simulink model "simulation_Hippocampus_compare_paper"  (R2023a)
settings: Solver=ode3  StartTime=0  StopTime=120  FixedStep=0.001  MaxStep=0.001  MinStep=0.00001  RelTol=1e-5  AbsTol=1e-5  EnableMultiTasking=on
values from neighbouring files (symbols this model uses):
  k_pos_ndi = 8    [parameters.m]
  k_vel_ndi = 8    [parameters.m]
  Kf = 6    [parameters.m]
  Kp = 0.01    [parameters.m]
  Kp_p = 30    [parameters.m]
  Kp_pitch = 8    [parameters.m]
  Kp_q = 10    [parameters.m]
  Kp_r = 10    [parameters.m]
  Kp_roll = 10    [parameters.m]
  Kp_u = 8    [parameters.m]
  Kp_yaw = 8    [parameters.m]
  Kq = 5    [parameters.m]
  Kr = 8    [parameters.m]
  Ktau1 = 0.1    [parameters.m]
  Ktau2 = 5    [parameters.m]
  Ktau3 = 5    [parameters.m]
  Ku = 8    [parameters.m]
  p11 = 0.4    [parameters.m]
  p12 = 0.2    [parameters.m]
  p21 = 0.2    [parameters.m]
  p22 = 0.05    [parameters.m]
  p31 = 0.3    [parameters.m]
  p32 = 0.05    [parameters.m]
  p41 = 0.5    [parameters.m]
  p42 = 0.1    [parameters.m]
  p51 = 0.5    [parameters.m]
  p52 = 0.1    [parameters.m]
  p61 = 0.5    [parameters.m]
  p62 = 0.1    [parameters.m]
  Q1 = -8    [simulation_para.m]
  Q2 = -10    [simulation_para.m]
  Q3 = -[0.01,5,8]    [simulation_para.m]
  Q4 = -[0.001,0.1,0.1]    [simulation_para.m]
  r1 = 4    [parameters.m]
  r2 = 6    [parameters.m]
libraries: simulink x8
(part 4 of 7)

== system simulation_Hippocampus_compare_paper/NDI4/Disturbance: All derivatives2/disturbance3/Subsystem1/wave frenquency ==
  Constant2 : Constant
  Constant3 : Constant  Value=1.1
  Constant4 : Constant  Value=1.2
  Constant5 : Constant  Value=0.5
  Constant6 : Constant  Value=0.6
  Constant7 : Constant  Value=0.7
  Mux : Mux  Inputs=6
  Out1 : Outport
  wires:
  Constant3/1 -> Mux/2
  Constant2/1 -> Mux/1
  Constant4/1 -> Mux/3
  Constant7/1 -> Mux/6
  Mux/1 -> Out1/1
  Constant5/1 -> Mux/4
  Constant6/1 -> Mux/5

== system simulation_Hippocampus_compare_paper/NDI4/Disturbance: All derivatives2/disturbance3/Subsystem1/wave percentage ==
  Constant{2..7} (6 alike) : Constant  Value=0
  Mux : Mux  Inputs=6
  Out1 : Outport
  wires:
  Constant3/1 -> Mux/2
  Constant2/1 -> Mux/1
  Constant4/1 -> Mux/3
  Constant7/1 -> Mux/6
  Mux/1 -> Out1/1
  Constant5/1 -> Mux/4
  Constant6/1 -> Mux/5

== system simulation_Hippocampus_compare_paper/PDPD/Disturbance: All derivatives1/disturbance3/Subsystem1/wave frenquency ==
  Constant2 : Constant
  Constant3 : Constant  Value=1.1
  Constant4 : Constant  Value=1.2
  Constant5 : Constant  Value=0.5
  Constant6 : Constant  Value=0.6
  Constant7 : Constant  Value=0.7
  Mux : Mux  Inputs=6
  Out1 : Outport
  wires:
  Constant3/1 -> Mux/2
  Constant2/1 -> Mux/1
  Constant4/1 -> Mux/3
  Constant7/1 -> Mux/6
  Mux/1 -> Out1/1
  Constant5/1 -> Mux/4
  Constant6/1 -> Mux/5

== system simulation_Hippocampus_compare_paper/PDPD/Disturbance: All derivatives1/disturbance3/Subsystem1/wave percentage ==
  Constant{2..7} (6 alike) : Constant  Value=0
  Mux : Mux  Inputs=6
  Out1 : Outport
  wires:
  Constant3/1 -> Mux/2
  Constant2/1 -> Mux/1
  Constant4/1 -> Mux/3
  Constant7/1 -> Mux/6
  Mux/1 -> Out1/1
  Constant5/1 -> Mux/4
  Constant6/1 -> Mux/5

== system simulation_Hippocampus_compare_paper/PDPD1/Disturbance: All derivatives1/disturbance3/Subsystem1/wave frenquency ==
  Constant2 : Constant
  Constant3 : Constant  Value=1.1
  Constant4 : Constant  Value=1.2
  Constant5 : Constant  Value=0.5
  Constant6 : Constant  Value=0.6
  Constant7 : Constant  Value=0.7
  Mux : Mux  Inputs=6
  Out1 : Outport
  wires:
  Constant3/1 -> Mux/2
  Constant2/1 -> Mux/1
  Constant4/1 -> Mux/3
  Constant7/1 -> Mux/6
  Mux/1 -> Out1/1
  Constant5/1 -> Mux/4
  Constant6/1 -> Mux/5

== system simulation_Hippocampus_compare_paper/PDPD1/Disturbance: All derivatives1/disturbance3/Subsystem1/wave percentage ==
  Constant{2..7} (6 alike) : Constant  Value=0
  Mux : Mux  Inputs=6
  Out1 : Outport
  wires:
  Constant3/1 -> Mux/2
  Constant2/1 -> Mux/1
  Constant4/1 -> Mux/3
  Constant7/1 -> Mux/6
  Mux/1 -> Out1/1
  Constant5/1 -> Mux/4
  Constant6/1 -> Mux/5

== system simulation_Hippocampus_compare_paper/Proposed Linear gain/Disturbance: All derivatives1/disturbance3/Subsystem1/wave frenquency ==
  Constant2 : Constant
  Constant3 : Constant  Value=1.1
  Constant4 : Constant  Value=1.2
  Constant5 : Constant  Value=0.5
  Constant6 : Constant  Value=0.6
  Constant7 : Constant  Value=0.7
  Mux : Mux  Inputs=6
  Out1 : Outport
  wires:
  Constant3/1 -> Mux/2
  Constant2/1 -> Mux/1
  Constant4/1 -> Mux/3
  Constant7/1 -> Mux/6
  Mux/1 -> Out1/1
  Constant5/1 -> Mux/4
  Constant6/1 -> Mux/5

== system simulation_Hippocampus_compare_paper/Proposed Linear gain/Disturbance: All derivatives1/disturbance3/Subsystem1/wave percentage ==
  Constant{2..7} (6 alike) : Constant  Value=0
  Mux : Mux  Inputs=6
  Out1 : Outport
  wires:
  Constant3/1 -> Mux/2
  Constant2/1 -> Mux/1
  Constant4/1 -> Mux/3
  Constant7/1 -> Mux/6
  Mux/1 -> Out1/1
  Constant5/1 -> Mux/4
  Constant6/1 -> Mux/5

== system simulation_Hippocampus_compare_paper/Proposed Linear gain/Disturbance: All derivatives2/disturbance3/Subsystem1/wave frenquency ==
  Constant2 : Constant
  Constant3 : Constant  Value=1.1
  Constant4 : Constant  Value=1.2
  Constant5 : Constant  Value=0.5
  Constant6 : Constant  Value=0.6
  Constant7 : Constant  Value=0.7
  Mux : Mux  Inputs=6
  Out1 : Outport
  wires:
  Constant3/1 -> Mux/2
  Constant2/1 -> Mux/1
  Constant4/1 -> Mux/3
  Constant7/1 -> Mux/6
  Mux/1 -> Out1/1
  Constant5/1 -> Mux/4
  Constant6/1 -> Mux/5

== system simulation_Hippocampus_compare_paper/Proposed Linear gain/Disturbance: All derivatives2/disturbance3/Subsystem1/wave percentage ==
  Constant{2..7} (6 alike) : Constant  Value=0
  Mux : Mux  Inputs=6
  Out1 : Outport
  wires:
  Constant3/1 -> Mux/2
  Constant2/1 -> Mux/1
  Constant4/1 -> Mux/3
  Constant7/1 -> Mux/6
  Mux/1 -> Out1/1
  Constant5/1 -> Mux/4
  Constant6/1 -> Mux/5

== system simulation_Hippocampus_compare_paper/Proposed Linear gain1/Disturbance: All derivatives1/disturbance3/Subsystem1/wave frenquency ==
  Constant2 : Constant
  Constant3 : Constant  Value=1.1
  Constant4 : Constant  Value=1.2
  Constant5 : Constant  Value=0.5
  Constant6 : Constant  Value=0.6
  Constant7 : Constant  Value=0.7
  Mux : Mux  Inputs=6
  Out1 : Outport
  wires:
  Constant3/1 -> Mux/2
  Constant2/1 -> Mux/1
  Constant4/1 -> Mux/3
  Constant7/1 -> Mux/6
  Mux/1 -> Out1/1
  Constant5/1 -> Mux/4
  Constant6/1 -> Mux/5

== system simulation_Hippocampus_compare_paper/Proposed Linear gain1/Disturbance: All derivatives1/disturbance3/Subsystem1/wave percentage ==
  Constant{2..7} (6 alike) : Constant  Value=0
  Mux : Mux  Inputs=6
  Out1 : Outport
  wires:
  Constant3/1 -> Mux/2
  Constant2/1 -> Mux/1
  Constant4/1 -> Mux/3
  Constant7/1 -> Mux/6
  Mux/1 -> Out1/1
  Constant5/1 -> Mux/4
  Constant6/1 -> Mux/5

== system simulation_Hippocampus_compare_paper/Proposed nonlinear gain/Disturbance: All derivatives1/disturbance3/Subsystem1/wave frenquency ==
  Constant2 : Constant
  Constant3 : Constant  Value=1.1
  Constant4 : Constant  Value=1.2
  Constant5 : Constant  Value=0.5
  Constant6 : Constant  Value=0.6
  Constant7 : Constant  Value=0.7
  Mux : Mux  Inputs=6
  Out1 : Outport
  wires:
  Constant3/1 -> Mux/2
  Constant2/1 -> Mux/1
  Constant4/1 -> Mux/3
  Constant7/1 -> Mux/6
  Mux/1 -> Out1/1
  Constant5/1 -> Mux/4
  Constant6/1 -> Mux/5

== system simulation_Hippocampus_compare_paper/Proposed nonlinear gain/Disturbance: All derivatives1/disturbance3/Subsystem1/wave percentage ==
  Constant{2..7} (6 alike) : Constant  Value=0
  Mux : Mux  Inputs=6
  Out1 : Outport
  wires:
  Constant3/1 -> Mux/2
  Constant2/1 -> Mux/1
  Constant4/1 -> Mux/3
  Constant7/1 -> Mux/6
  Mux/1 -> Out1/1
  Constant5/1 -> Mux/4
  Constant6/1 -> Mux/5

== system simulation_Hippocampus_compare_paper/Proposed nonlinear gain1/Disturbance: All derivatives1/disturbance3/Subsystem1/wave frenquency ==
  Constant2 : Constant
  Constant3 : Constant  Value=1.1
  Constant4 : Constant  Value=1.2
  Constant5 : Constant  Value=0.5
  Constant6 : Constant  Value=0.6
  Constant7 : Constant  Value=0.7
  Mux : Mux  Inputs=6
  Out1 : Outport
  wires:
  Constant3/1 -> Mux/2
  Constant2/1 -> Mux/1
  Constant4/1 -> Mux/3
  Constant7/1 -> Mux/6
  Mux/1 -> Out1/1
  Constant5/1 -> Mux/4
  Constant6/1 -> Mux/5

== system simulation_Hippocampus_compare_paper/Proposed nonlinear gain1/Disturbance: All derivatives1/disturbance3/Subsystem1/wave percentage ==
  Constant{2..7} (6 alike) : Constant  Value=0
  Mux : Mux  Inputs=6
  Out1 : Outport
  wires:
  Constant3/1 -> Mux/2
  Constant2/1 -> Mux/1
  Constant4/1 -> Mux/3
  Constant7/1 -> Mux/6
  Mux/1 -> Out1/1
  Constant5/1 -> Mux/4
  Constant6/1 -> Mux/5

== matlab function simulation_Hippocampus_compare_paper/Proposed Linear gain1/HippCampus/Subsystem1/norm1 ==
  data: u input; y output
function y  = fcn(u)
y=norm(u)^2;
end

== matlab function simulation_Hippocampus_compare_paper/Proposed Linear gain1/HippCampus/Subsystem4/Subsystem/norm1 ==
  data: u input; y output
function y  = fcn(u)
y=norm(u)^2;
end

== matlab function simulation_Hippocampus_compare_paper/Proposed Linear gain1/HippCampus/Subsystem4/Subsystem1/norm1 ==
  data: u input; y output
function y  = fcn(u)
y=norm(u)^2;
end

== matlab function simulation_Hippocampus_compare_paper/Proposed Linear gain1/HippCampus/Subsystem4/Subsystem2/norm1 ==
  data: u input; y output
function y  = fcn(u)
y=norm(u)^2;
end

== matlab function simulation_Hippocampus_compare_paper/Proposed Linear gain1/HippCampus/Subsystem4/Subsystem3/norm1 ==
  data: u input; y output
function y  = fcn(u)
y=norm(u)^2;
end

== matlab function simulation_Hippocampus_compare_paper/Proposed nonlinear gain1/Controller/MATLAB Function1 ==
  data: ref input; K output; s input; k input; parameter input
%---------------------------------------------------------------------------------------------
% For Paper, 
% "Three-Dimensional Simultaneous Stabilization and Tracking Control of Nonholonomic Autonomous Underwater Vehicles"
% by Shuyuan Fan and Herbert Werner
% Copyright (c) Institute of Control Systems, Hamburg University of Technology. All rights reserved.
% Licensed under the GPLv3. See LICENSE in the project root for license information.
% Uses an own implementation of the work of 
% IEEE Conference on Decision and Control and L-CSS, 2022."
% Author(s): Shuyuan Fan
%--------------------------------------------------------------------------------------------
function K= fcn(ref,s,k,parameter)


%% reference
x_ref = ref(1);y_ref = ref(2);z_ref = ref(3);

%% states
x = s(1);y = s(2);z = s(3);
phi = s(4); phi =min(max(phi,-0.5),0.5);
theta = s(5); 
theta = min(max(theta,-1.5),1.5);
psi = s(6); psi =  wrapToPi(psi);
u=s(7);v=s(8);w=s(9); p =s(10);
q=s(11);r=s(12);

%% error
e_x = x_ref-x;
e_y = y_ref - y;
e_z = z_ref - z;

%% design attitude trajectory
psi_des = atan2(e_y, e_x);
e_psi = psi_des -psi;
e_psi = atan2(sin(e_psi), cos(e_psi));

theta_des = -atan2(e_z,(e_x^2+e_y^2)^0.5);
theta_des = min(max(theta_des,-1.5),1.5);
e_theta = theta_des - theta;

e_phi=0-phi;

%% gain
K0 =k(1);
K1 =k(2);
K2 =k(3);
K3 =k(4);

%% nonlinear gain
a1 = e_x^2 + e_y^2 + e_z^2;
a2=(e_x^2+e_y^2)^0.5;
p11 = parameter(1);
p12 = parameter(2);
p21 = parameter(3);
p22 = parameter(4);
p31 = parameter(5);
p32 = parameter(6);
e1 = e_x*cos(theta)*cos(psi)+e_y*cos(theta)*sin(psi)-e_z * sin(theta);
K0 = K0*(sqrt(a1)+p11)/(sqrt(a1)+p12);
K2 = K2*(abs(e_theta)+p21)/(abs(e_theta)+p22);
K3 = K3*(1*abs(e_psi)+p31)/(abs(e_psi)+p32);

% K0 = K0*(sqrt(a1)+0.4)/(sqrt(a1)+0.1);
% K2 = K2*(abs(e_theta)+0.2)/(abs(e_theta)+0.1);
% K3 = K3*(1*abs(e_psi)+0.5)/(abs(e_psi)+0.2);

%% design u

ud = K0*e1;

%% calculate exdot,eydot,ezdot

R =- [  cos(psi)*cos(theta)  cos(psi)*sin(theta)*sin(phi)-sin(psi)*cos(phi)  cos(psi)*cos(phi)*sin(theta)+sin(psi)*sin(phi) ;
           sin(psi)*cos(theta)  sin(psi)*sin(theta)*sin(phi)+cos(psi)*cos(phi)  sin(psi)*cos(phi)*sin(theta)-cos(psi)*sin(phi) ;
          -sin(theta)           cos(theta)*sin(phi)                             cos(theta)*cos(phi)                            ];

ee=R*[u;v;w];
exdot=ee(1);
eydot=ee(2);
ezdot=ee(3);


%% calculate theta_d_dot psi_d_dot
% % because atan2 is not continued and its derivative is not existing 
if abs(e_x)+abs(e_y)==0
%if  norm(e_x)+ norm(e_y) + norm(e_z) ==0 || norm(e_x)+ norm(e_y)==0
  theta_des_dot =0;
else
    theta_des_dot= -(ezdot*a2^2-2*e_z*(e_x*exdot+e_y*eydot))/(a1*a2+eps);
end

if abs(e_x)+abs(e_y)==0
    psi_des_dot = 0;
else
   psi_des_dot = (eydot*(e_x)-exdot*e_y)/((e_x)^2+e_y^2+eps);
end

 theta_des_dot = min(max(theta_des_dot,-3),3);
 psi_des_dot = min(max(psi_des_dot,-3),3);


%% design pd qd rd

pd = K1*e_phi-sin(phi)*tan(theta)*q-cos(phi)*tan(theta)*r;
qd = (K2*e_theta +r*sin(phi)+theta_des_dot)/(cos(phi)+eps);
rd = cos(theta)/(cos(phi)+eps)*(K3*e_psi+1*psi_des_dot-q*sin(phi)/(cos(theta)+eps));


%% saturation 
% ud=min(max(ud,-10),10);
% pd=min(max(pd,-6),6);
% qd=min(max(qd,-6),6);
% rd=min(max(rd,-10),10);

K = [ud;pd;qd;rd;e1;e_phi;e_theta;e_psi;theta_des_dot;psi_des_dot];
end

== matlab function simulation_Hippocampus_compare_paper/Stabilizing without v w /Controller/Kinematic1 ==
  data: sd input; s input; output output; sd_dot input; error1 input; k2 input
%---------------------------------------------------------------------------------------------
% For Paper, 
% "Three-Dimensional Simultaneous Stabilization and Tracking Control of Nonholonomic Autonomous Underwater Vehicles"
% by Shuyuan Fan and Herbert Werner
% Copyright (c) Institute of Control Systems, Hamburg University of Technology. All rights reserved.
% Licensed under the GPLv3. See LICENSE in the project root for license information.
% Uses an own implementation of the work of 
% IEEE Conference on Decision and Control and L-CSS, 2022."
% Author(s): Shuyuan Fan
%--------------------------------------------------------------------------------------------
function output = fcn(sd,s,sd_dot,error1,k2)  
    zg    =  0.05;    % [m]
    g     =  9.81;    % [m/s^2]

    m     =  1.43;    % [kg]
    Ix    = 0.00241; % [kgm^2]
    Iy    = 0.01072; % [kgm^2]
    Iz    = 0.01072; % [kgm^2]
    Xudot = -1.11;    % [kg]
    Yvdot = -2.80;    % [kg]
    Zwdot = -2.80;    % [kg]
    Kpdot = -0.0018;  % [kgm^2]
    Mqdot = -0.0095;  % [kgm^2]
    Nrdot = -0.0095;  % [kgm^2]
    Xu    = -4.56;    % [kg/m]
    Yv    = -17.36;   % [kg/m]
    Zw    = -17.36;   % [kg/m]
    Kp    = -0.0028;  % [kgm^2]
    Mq    = -0.0476;  % [kgm^2]
    Nr    = -0.0476;  % [kgm^2]

    udes = sd(1); pdes = sd(2);qdes=sd(3);rdes=sd(4);
    x=s;
    
    udes_dot=sd_dot(1);pd_dot =sd_dot(2);qd_dot = sd_dot(3);
    rd_dot = sd_dot(4); 
    
    e1 = error1(1);e_phi = error1(2);e_theta= error1(3);
    e_psi = error1(4);

    % Extract states into more readable form
    phi = x( 4); theta = x(5); psi = x( 6);
    u   = x( 7); v     = x( 8); w   = x( 9);
    p   = x(10); q     = x(11); r   = x(12);
    nu  = x(7:12);
    theta = min(max(theta,-1.5),1.5);
    % Construct rotational tensor
  R = [  cos(psi)*cos(theta)  cos(psi)*sin(theta)*sin(phi)-sin(psi)*cos(phi)  cos(psi)*cos(phi)*sin(theta)+sin(psi)*sin(phi) ;
   sin(psi)*cos(theta)  sin(psi)*sin(theta)*sin(phi)+cos(psi)*cos(phi)  sin(psi)*cos(phi)*sin(theta)-cos(psi)*sin(phi) ;
  -sin(theta)           cos(theta)*sin(phi)                            cos(theta)*cos(phi)                            ];


    % Construct velocity transformation tensor
    T = [ 1  sin(phi)*tan(theta)   cos(phi)*tan(theta) ;
          0  cos(phi)             -sin(phi)            ;
          0  sin(phi)/cos(theta)   cos(phi)/cos(theta) ];
    J = blkdiag(R, T);

    % Calculate mass matrix
    Ma  = -blkdiag(Xudot, Yvdot, Zwdot, Kpdot, Mqdot, Nrdot);
    Mrb =  blkdiag(eye(3) * m, Ix, Iy, Iz);
    M = Ma + Mrb;

    % Compute hydrostatic load
    gravity = zg * g * m;
    G = blkdiag(0,0,0, gravity * cos(theta) * (sin(phi)/(phi+eps)), gravity * (sin(theta)/(theta+eps)), 0);

    % Construct coriolis matrix, see Fossen 2011, Theorem 3.2
    C = [  zeros(3)                    -skew(M(1:3,1:3) * nu(1:3)) ;
          -skew(M(1:3,1:3) * nu(1:3))  -skew(M(4:6,4:6) * nu(4:6)) ];

    % Construct damping matrix
    D = -blkdiag(Xu * abs(u), Yv * abs(v),...
                 Zw * abs(w), Kp * abs(p),...
                 Mq * abs(q), Nr * abs(r));

    % Build state space equations
    
    Mi  = inv(M);
    A   = [ zeros(6), J; -Mi*G, -Mi*(C+D) ];
     
    dx  = A * x ;
    udot = dx(7);
    pdot = dx(10);
    qdot = dx(11);
    rdot = dx(12);
    
%%gain   

Kf =k2(1);
K_t1 =k2(2);
K_t2 =k2(3);
K_t3 =k2(4);


%% error2
eu = udes-u;
ep =pdes-p;
eq = qdes-q;
er = rdes-r;


%% nonlinear gain
% Kf=(1*abs(eu)+0.4)/(1*abs(eu)+0.11)*Kf;
% %K_t1 = (1*abs(ep)+0.15)/(1*abs(ep)+0.1)*K_t1;
% K_t2 = (1*abs(eq)+0.5)/(1*abs(eq)+0.1)*K_t2;
% K_t3 = (1*abs(er)+0.5)/(1*abs(er)+0.1)*K_t3;



%% controller
f=Kf*eu-udot*(m-Xudot)+udes_dot*(m-Xudot)+(m-Xudot)*e1;
tau1 = K_t1 * ep+0*(Ix-Kpdot)*(e_phi+pd_dot-pdot);
tau2 = K_t2 * eq  +(qd_dot+cos(phi)*e_theta-qdot)*(Iy-Mqdot);
tau3 = K_t3* er +(rd_dot+cos(phi)/(cos(theta)+eps)*e_psi-rdot)*(Iz-Nrdot);

controller =  [f;tau1;tau2;tau3];
error2 =[eu;ep;eq;er];

output = [controller;error2];



   

end
function S = skew(lambda)
    S = [  0          -lambda(3)   lambda(2) ;
           lambda(3)   0          -lambda(1) ;
          -lambda(2)   lambda(1)   0         ]; 
end

== matlab function simulation_Hippocampus_compare_paper/Proposed Linear gain1/norm ==
  data: u input; y output
function y  = fcn(u)
y=norm(u)^2;
end

== matlab function simulation_Hippocampus_compare_paper/Proposed Linear gain1/norm1 ==
  data: u input; y output
function y  = fcn(u)
y=norm(u);
end

== matlab function simulation_Hippocampus_compare_paper/Proposed nonlinear gain1/Controller/calculate derivative 1/MATLAB Function ==
  data: u input; y output; t input
function y = fcn(u,t)
if t>0.1
    y=u;
else
    y=[0;0;0;0];
end

== matlab function simulation_Hippocampus_compare_paper/Proposed nonlinear gain1/Disturbance: All derivatives1/MATLAB Function ==
  data: u input; y output; d input
function y = fcn(u,d)

y = u*d;

== matlab function simulation_Hippocampus_compare_paper/Proposed nonlinear gain1/Disturbance: All derivatives1/disturbance3/MATLAB Function ==
  data: p input; a input; d output; u_wave input; u_c input; u_un input
%% wind disturbance, wave disturbance, ocean currents and modeling uncertainties(Fossen 2011)
%for AUV, we can neglect the wind disturbance
%wave disturbance is in R^6
%Ocean Currents are related to the hydrodynamic terms. Here we consider
%them as the friction forces 
%modeling uncertainties can be assumed as constant terms
%assume all disturbances are constant
function d = fcn(p,a,u_wave, u_c,u_un)
%a: attitude states
%u_wave: parameters of u_wave
%u_c ocean currents percentage
%u_un uncertainty percentage
%ocean currents
phi=a(1);
theta=a(2);
psi = a(3);
V = u_c(1)/100*4.724; % 0<V<4.724
theta_c=u_c(2);
psi_c = u_c(3);
 R = [  cos(psi)*cos(theta)  cos(psi)*sin(theta)*sin(phi)-sin(psi)*cos(phi)  cos(psi)*cos(phi)*sin(theta)+sin(psi)*sin(phi) ;
           sin(psi)*cos(theta)  sin(psi)*sin(theta)*sin(phi)+cos(psi)*cos(phi)  sin(psi)*cos(phi)*sin(theta)-cos(psi)*sin(phi) ;
          -sin(theta)           cos(theta)*sin(phi)                             cos(theta)*cos(phi)                            ];
uc=[V*cos(theta_c)*cos(psi_c);V*sin(psi_c);V*sin(theta_c)*cos(psi_c)];
f_c=R*uc;
d_c=[f_c;zeros(3,1)];

%wave disturbance
k1=u_wave(1:6); %amplitude 
k2 = u_wave(7:12); %frequency 
time=u_wave(13);
d_w = [k1(1)/100*4.724*sin(k2(1)*time);k1(2)/100*4.724*sin(k2(2)*time);k1(3)/100*4.724*sin(k2(3)*time);
    k1(4)/100*6.841*sin(k2(4)*time);k1(5)/100*28.55*sin(k2(5)*time);k1(6)/100*28.55*sin(k2(6)*time)];
%model uncertainties
%u_un uncertainty percentage
d_u=u_un/100*[4.724;0;0;6.841;28.55;28.55];

x=p(1);
y=p(2);
z=p(3);
if y>2 && y<2.5 || y<-2 && y>-2.5
    tau_d=d_c+d_w+d_u;
else
    tau_d=zeros(6,1);
end
    
d=[zeros(6,1);tau_d];

== matlab function simulation_Hippocampus_compare_paper/Proposed nonlinear gain1/HippCampus/HippoCampus ==
  data: x input; dx output; in input
function dx = fcn(x, in)
zg    =  0.05;    % [m]
g     =  9.81;    % [m/s^2]

m     =  1.43;    % [kg]
Ix    = 0.00241; % [kgm^2]
Iy    = 0.01072; % [kgm^2]
Iz    = 0.01072; % [kgm^2]
Xudot = -1.11;    % [kg]
Yvdot = -2.80;    % [kg]
Zwdot = -2.80;    % [kg]
Kpdot = -0.0018;  % [kgm^2]
Mqdot = -0.0095;  % [kgm^2]
Nrdot = -0.0095;  % [kgm^2]
Xu    = -4.56;    % [kg/m]
Yv    = -17.36;   % [kg/m]
Zw    = -17.36;   % [kg/m]
Kp    = -0.0028;  % [kgm^2]
Mq    = -0.0476;  % [kgm^2]
Nr    = -0.0476;  % [kgm^2]
% Extract states into more readable form
phi = x( 4); theta = x( 5);
u   = x( 7); v     = x( 8); w   = x( 9);
p   = x(10); q     = x(11); r   = x(12);
nu  = x(7:12);
% Construct rotational tensor
R = body_frame_rotation(x(4:6));

% Construct velocity transformation tensor
T = [ 1  sin(phi)*tan(theta)   cos(phi)*tan(theta) ;
    0  cos(phi)             -sin(phi)            ;
    0  sin(phi)/cos(theta)   cos(phi)/cos(theta) ];
J = [ R         zeros(3) ;
    zeros(3)  T        ];

% Calculate mass matrix
Ma  = -diag([Xudot, Yvdot, Zwdot, Kpdot, Mqdot, Nrdot]);
Mrb =  diag([m,  m,  m, Ix, Iy, Iz]);
M = Ma + Mrb;

% Compute hydrostatic load
gravity = zg * g * m;
G = [ 0; 0; 0; gravity * cos(theta) * sin(phi); gravity * sin(theta); 0 ];

% Construct coriolis matrix, see Fossen 2011, Theorem 3.2
C12 = -skew(M(1:3,1:3) * nu(1:3));
C = [ zeros(3)   C12                        ;
    C12       -skew(M(4:6,4:6) * nu(4:6)) ];

% Construct damping matrix
D = -diag([Xu * abs(u), Yv * abs(v),...
    Zw * abs(w), Kp * abs(p),...
    Mq * abs(q), Nr * abs(r)]);

% Build state space equations
tau  = [ in(1); 0; 0; in(2:4) ];

dx       = zeros(12,1);
dx(1:6)  = J*nu;
dx(7:12) = M \ (tau - (C+D)*nu - G);
end

function S = skew(lambda)
S = [  0          -lambda(3)   lambda(2) ;
    lambda(3)   0          -lambda(1) ;
    -lambda(2)   lambda(1)   0         ];
end

function R = body_frame_rotation(Phi)
phi = Phi(1); theta = Phi(2); psi = Phi(3);

R = [  cos(psi)*cos(theta)  cos(psi)*sin(theta)*sin(phi)-sin(psi)*cos(phi)  cos(psi)*cos(phi)*sin(theta)+sin(psi)*sin(phi) ;
    sin(psi)*cos(theta)  sin(psi)*sin(theta)*sin(phi)+cos(psi)*cos(phi)  sin(psi)*cos(phi)*sin(theta)-cos(psi)*sin(phi) ;
    -sin(theta)           cos(theta)*sin(phi)                             cos(theta)*cos(phi)                            ];
end

== matlab function simulation_Hippocampus_compare_paper/Proposed nonlinear gain1/HippCampus/Subsystem/MATLAB Function ==
  data: u input; y output
function y = fcn(u)
y =  wrapToPi(u);

== matlab function simulation_Hippocampus_compare_paper/Proposed nonlinear gain1/HippCampus/Subsystem1/norm1 ==
  data: u input; y output
function y  = fcn(u)
y=norm(u)^2;
end

== matlab function simulation_Hippocampus_compare_paper/Proposed nonlinear gain1/HippCampus/Subsystem4/Subsystem/norm1 ==
  data: u input; y output
function y  = fcn(u)
y=norm(u)^2;
end

== matlab function simulation_Hippocampus_compare_paper/Proposed nonlinear gain1/HippCampus/Subsystem4/Subsystem1/norm1 ==
  data: u input; y output
function y  = fcn(u)
y=norm(u)^2;
end

== matlab function simulation_Hippocampus_compare_paper/Proposed nonlinear gain1/HippCampus/Subsystem4/Subsystem2/norm1 ==
  data: u input; y output
function y  = fcn(u)
y=norm(u)^2;
end

== matlab function simulation_Hippocampus_compare_paper/Proposed nonlinear gain1/HippCampus/Subsystem4/Subsystem3/norm1 ==
  data: u input; y output
function y  = fcn(u)
y=norm(u)^2;
end

== matlab function simulation_Hippocampus_compare_paper/Proposed nonlinear gain2/Controller/Passive Sigma2 ==
  data: s input; nu_f input; f output; Q2 input
%---------------------------------------------------------------------------------------------
% For Paper, 
% "Three-Dimensional Simultaneous Stabilization and Tracking Control of Nonholonomic Autonomous Underwater Vehicles"
% by Shuyuan Fan and Herbert Werner
% Copyright (c) Institute of Control Systems, Hamburg University of Technology. All rights reserved.
% Licensed under the GPLv3. See LICENSE in the project root for license information.
% Uses an own implementation of the work of 
% IEEE Conference on Decision and Control and L-CSS, 2022."
% Author(s): Shuyuan Fan
%--------------------------------------------------------------------------------------------
function f= fcn(s,nu_f,Q2)
zg    =  0.05;    % [m]
g     =  9.81;    % [m/s^2]

m     =  1.43;    % [kg]
Ix    = 0.00241; % [kgm^2]
Iy    = 0.01072; % [kgm^2]
Iz    = 0.01072; % [kgm^2]
Xudot = -1.11;    % [kg]
Yvdot = -2.80;    % [kg]
Zwdot = -2.80;    % [kg]
Kpdot = -0.0018;  % [kgm^2]
Mqdot = -0.0095;  % [kgm^2]
Nrdot = -0.0095;  % [kgm^2]
Xu    = -4.56;    % [kg/m]
Yv    = -17.36;   % [kg/m]
Zw    = -17.36;   % [kg/m]
Kp    = -0.0028;  % [kgm^2]
Mq    = -0.0476;  % [kgm^2]
Nr    = -0.0476;  % [kgm^2]

% Calculate mass matrix
Ma  = -diag([Xudot, Yvdot, Zwdot, Kpdot, Mqdot, Nrdot]);
Mrb =  diag([m,  m,  m, Ix, Iy, Iz]);
M = Ma + Mrb;

M1 = M(1:3,1:3);




%% states
x = s(1); y = s(2); z = s(3);
X = s(1:3);

angle = s(4:6);
phi = s(4);
%phi =min(max(phi,-0.5),0.5);
theta = s(5); 
%theta = min(max(theta,-1.5),1.5);
psi = s(6);
%psi =  wrapToPi(psi);
nu = s(7:9) ;
u=s(7); v=s(8); w=s(9); 

omega = s(10:12);
p=s(10); q=s(11); r=s(12);


% Gamma function for nu
Gamma_nu = vectortodirect(nu);

y2 = u/Gamma_nu(1);
y2star = y2 - nu_f;
% storage function V2
V2 = 0.5*y2star'*Gamma_nu'*M1*M1*Gamma_nu*y2star;


C1 = -skew(M(1:3,1:3) * nu);
D = -diag([Xu * abs(u), Yv * abs(v),...
    Zw * abs(w), Kp * abs(p),...
    Mq * abs(q), Nr * abs(r)]);
D1 = D(1:3,1:3);
H = -C1*omega-D1*nu;

Gamma_0 = [1;0;0];
f = (Q2*y2star - H'*M1*Gamma_nu)/(Gamma_0'*M1*Gamma_nu);

%% Theta_d

end

== matlab function simulation_Hippocampus_compare_paper/Proposed nonlinear gain1/norm ==
  data: u input; y output
function y  = fcn(u)
y=norm(u)^2;
end

== matlab function simulation_Hippocampus_compare_paper/Proposed nonlinear gain1/norm1 ==
  data: u input; y output
function y  = fcn(u)
y=norm(u);
end

== matlab function simulation_Hippocampus_compare_paper/PDPD/HippCampus1/Subsystem/MATLAB Function ==
  data: u input; y output
function y = fcn(u)
y =  wrapToPi(u);

== matlab function simulation_Hippocampus_compare_paper/Stabilizing without v w 1/Controller/Kinematic1 ==
  data: s input; output output
%---------------------------------------------------------------------------------------------
% For Paper, 
% "Three-Dimensional Simultaneous Stabilization and Tracking Control of Nonholonomic Autonomous Underwater Vehicles"
% by Shuyuan Fan and Herbert Werner
% Copyright (c) Institute of Control Systems, Hamburg University of Technology. All rights reserved.
% Licensed under the GPLv3. See LICENSE in the project root for license information.
% Uses an own implementation of the work of 
% IEEE Conference on Decision and Control and L-CSS, 2022."
% Author(s): Shuyuan Fan
%--------------------------------------------------------------------------------------------
function output = fcn(s)  
    zg    =  0.05;    % [m]
    g     =  9.81;    % [m/s^2]

    m     =  1.43;    % [kg]
    Ix    = 0.00241; % [kgm^2]
    Iy    = 0.01072; % [kgm^2]
    Iz    = 0.01072; % [kgm^2]
    Xudot = -1.11;    % [kg]
    Yvdot = -2.80;    % [kg]
    Zwdot = -2.80;    % [kg]
    Kpdot = -0.0018;  % [kgm^2]
    Mqdot = -0.0095;  % [kgm^2]
    Nrdot = -0.0095;  % [kgm^2]
    Xu    = -4.56;    % [kg/m]
    Yv    = -17.36;   % [kg/m]
    Zw    = -17.36;   % [kg/m]
    Kp    = -0.0028;  % [kgm^2]
    Mq    = -0.0476;  % [kgm^2]
    Nr    = -0.0476;  % [kgm^2]
    udes = s(1); pdes = s(2);qdes=s(3);rdes=s(4);
    x=s(5:16);udes_dot=s(17);pd_dot =s(18);qd_dot = s(19);
    rd_dot = s(20);e1 = s(21);e_phi = s(22);e_theta= s(23);
    e_psi = s(24);
    % Extract states into more readable form
    phi = x( 4); theta = x(5); psi = x( 6);
    u   = x( 7); v     = x( 8); w   = x( 9);
    p   = x(10); q     = x(11); r   = x(12);
    nu  = x(7:12);
    theta = min(max(theta,-1.5),1.5);

    % Construct rotational tensor
  R = [  cos(psi)*cos(theta)  cos(psi)*sin(theta)*sin(phi)-sin(psi)*cos(phi)  cos(psi)*cos(phi)*sin(theta)+sin(psi)*sin(phi) ;
   sin(psi)*cos(theta)  sin(psi)*sin(theta)*sin(phi)+cos(psi)*cos(phi)  sin(psi)*cos(phi)*sin(theta)-cos(psi)*sin(phi) ;
  -sin(theta)           cos(theta)*sin(phi)                            cos(theta)*cos(phi)                            ];


    % Construct velocity transformation tensor
    T = [ 1  sin(phi)*tan(theta)   cos(phi)*tan(theta) ;
          0  cos(phi)             -sin(phi)            ;
          0  sin(phi)/cos(theta)   cos(phi)/cos(theta) ];
    J = blkdiag(R, T);

    % Calculate mass matrix
    Ma  = -blkdiag(Xudot, Yvdot, Zwdot, Kpdot, Mqdot, Nrdot);
    Mrb =  blkdiag(eye(3) * m, Ix, Iy, Iz);
    M = Ma + Mrb;

    % Compute hydrostatic load
    gravity = zg * g * m;
    G = blkdiag(0,0,0, gravity * cos(theta) * (sin(phi)/(phi+eps)), gravity * (sin(theta)/(theta+eps)), 0);

    % Construct coriolis matrix, see Fossen 2011, Theorem 3.2
    C = [  zeros(3)                    -skew(M(1:3,1:3) * nu(1:3)) ;
          -skew(M(1:3,1:3) * nu(1:3))  -skew(M(4:6,4:6) * nu(4:6)) ];

    % Construct damping matrix
    D = -blkdiag(Xu * abs(u), Yv * abs(v),...
                 Zw * abs(w), Kp * abs(p),...
                 Mq * abs(q), Nr * abs(r));

    % Build state space equations
    
    Mi  = inv(M);
    A   = [ zeros(6), J; -Mi*G, -Mi*(C+D) ];
     
    dx  = A * x ;
    udot = dx(7);
    pdot = dx(10);
    qdot = dx(11);
    rdot = dx(12);
    
   

Kf =8;
K_t1 =0.001;
K_t2 =2.0;
K_t3 =5;
eu = udes-u;
f=Kf*eu-udot*(m-Xudot)+udes_dot*(m-Xudot)+(m-Xudot)*e1;



ep =pdes-p;
eq = qdes-q;
er = rdes-r;


tau1 = K_t1 * ep+0*(Ix-Kpdot)*(e_phi+1*pd_dot-1*pdot);
tau2 = K_t2 * eq  +(1*qd_dot+cos(phi)*e_theta-qdot)*(Iy-Mqdot);
tau3 = K_t3* er +(1*rd_dot+cos(phi)/cos(theta)*e_psi-rdot)*(Iz-Nrdot);


output = [f;tau1;tau2;tau3];



   

end
function S = skew(lambda)
    S = [  0          -lambda(3)   lambda(2) ;
           lambda(3)   0          -lambda(1) ;
          -lambda(2)   lambda(1)   0         ]; 
end

== matlab function simulation_Hippocampus_compare_paper/Stabilizing without v w 1/Controller/MATLAB Function1 ==
  data: s input; K output
%---------------------------------------------------------------------------------------------
% For Paper, 
% "Three-Dimensional Simultaneous Stabilization and Tracking Control of Nonholonomic Autonomous Underwater Vehicles"
% by Shuyuan Fan and Herbert Werner
% Copyright (c) Institute of Control Systems, Hamburg University of Technology. All rights reserved.
% Licensed under the GPLv3. See LICENSE in the project root for license information.
% Uses an own implementation of the work of 
% IEEE Conference on Decision and Control and L-CSS, 2022."
% Author(s): Shuyuan Fan
%--------------------------------------------------------------------------------------------
function K= fcn(s)
x_ref = s(1);y_ref = s(2);z_ref = s(3);
x = s(4);y = s(5);z = s(6);
phi = s(7);phi =  wrapToPi(phi);
theta = s(8);theta =  wrapToPi(theta);
psi = s(9); psi =  wrapToPi(psi);
u=s(10);v=s(11);w=s(12);
q=s(14);r=s(15);
e_x = x_ref-x;
e_y = y_ref - y;
e_z = z_ref - z;

psi_des = atan2(e_y, e_x);
e_psi = psi_des -psi;
e_psi = atan2(sin(e_psi), cos(e_psi));

theta = min(max(theta,-1.5),1.5);
theta_des = -atan2(e_z,(e_x^2+e_y^2)^0.5);
theta_des = min(max(theta_des,-1.5),1.5);
e_theta = theta_des - theta;
K0 =8;
K1 =0.01;
K2 =2;
K3 =5;
%K2 = K2*(e_theta+0.5)/(1*e_theta+0.005);

a1 = e_x^2 + e_y^2 + e_z^2;
%K3 = K3*(a1+0.5)/(a1+0.02);


ud =K0*(e_x*cos(theta)*cos(psi)+e_y*cos(theta)*sin(psi)-e_z * sin(theta));
  e1 = e_x*cos(theta)*cos(psi)+e_y*cos(theta)*sin(psi)-e_z * sin(theta);
R =- [  cos(psi)*cos(theta)  cos(psi)*sin(theta)*sin(phi)-sin(psi)*cos(phi)  cos(psi)*cos(phi)*sin(theta)+sin(psi)*sin(phi) ;
           sin(psi)*cos(theta)  sin(psi)*sin(theta)*sin(phi)+cos(psi)*cos(phi)  sin(psi)*cos(phi)*sin(theta)-cos(psi)*sin(phi) ;
          -sin(theta)           cos(theta)*sin(phi)                             cos(theta)*cos(phi)                            ];

ee=R*[u;v;w];
exdot=ee(1);
eydot=ee(2);
ezdot=ee(3);
a2=(e_x^2+e_y^2)^0.5;


if  norm(e_x)+ norm(e_y) + norm(e_z) == 0 || norm(e_x)+ norm(e_y)==0
   theta_des_dot =0;
else
    theta_des_dot= -(ezdot*a2^2-2*e_z*(e_x*exdot+e_y*eydot))/(a1*a2);
end

if norm(e_x)+norm(e_y)==0
    psi_des_dot = 0;
else
   psi_des_dot = (eydot*(e_x)-exdot*e_y)/((e_x)^2+1*e_y^2);
end


pd = K1*(0-phi)-sin(phi)*tan(theta)*q-cos(phi)*tan(theta)*r;
qd = (K2*e_theta +r*sin(phi)+theta_des_dot)/cos(phi);
rd = cos(theta)/cos(phi)*(K3*e_psi+1*psi_des_dot-q*sin(phi)/cos(theta));
e_phi=0-phi;

%ud = 5*tanh(ud);
%pd = 5*tanh(pd);
%qd = 5*tanh(qd);
%rd = 5*tanh(rd);
ud=min(max(ud,-5),5);
pd=min(max(pd,-5),5);
qd=min(max(qd,-5),5);
rd=min(max(rd,-5),5);

K = [ud;pd;qd;rd;e1;e_phi;e_theta;e_psi];

== matlab function simulation_Hippocampus_compare_paper/Stabilizing without v w 1/Controller/calculate derivative /MATLAB Function ==
  data: u input; y output; t input
function y = fcn(u,t)
if t>0.1
    y=u;
else
    y=[0;0;0;0];
end

== matlab function simulation_Hippocampus_compare_paper/Stabilizing without v w 1/HippCampus/HippoCampus ==
  data: x input; dx output; in input
function dx = fcn(x, in)
zg    =  0.05;    % [m]
g     =  9.81;    % [m/s^2]

m     =  1.43;    % [kg]
Ix    = 0.00241; % [kgm^2]
Iy    = 0.01072; % [kgm^2]
Iz    = 0.01072; % [kgm^2]
Xudot = -1.11;    % [kg]
Yvdot = -2.80;    % [kg]
Zwdot = -2.80;    % [kg]
Kpdot = -0.0018;  % [kgm^2]
Mqdot = -0.0095;  % [kgm^2]
Nrdot = -0.0095;  % [kgm^2]
Xu    = -4.56;    % [kg/m]
Yv    = -17.36;   % [kg/m]
Zw    = -17.36;   % [kg/m]
Kp    = -0.0028;  % [kgm^2]
Mq    = -0.0476;  % [kgm^2]
Nr    = -0.0476;  % [kgm^2]
% Extract states into more readable form
phi = x( 4); theta = x( 5);
u   = x( 7); v     = x( 8); w   = x( 9);
p   = x(10); q     = x(11); r   = x(12);
nu  = x(7:12);
v =0;
w=0;
% Construct rotational tensor
R = body_frame_rotation(x(4:6));

% Construct velocity transformation tensor
T = [ 1  sin(phi)*tan(theta)   cos(phi)*tan(theta) ;
    0  cos(phi)             -sin(phi)            ;
    0  sin(phi)/cos(theta)   cos(phi)/cos(theta) ];
J = [ R         zeros(3) ;
    zeros(3)  T        ];

% Calculate mass matrix
Ma  = -diag([Xudot, Yvdot, Zwdot, Kpdot, Mqdot, Nrdot]);
Mrb =  diag([m,  m,  m, Ix, Iy, Iz]);
M = Ma + Mrb;

% Compute hydrostatic load
gravity = zg * g * m;
G = [ 0; 0; 0; gravity * cos(theta) * sin(phi); gravity * sin(theta); 0 ];

% Construct coriolis matrix, see Fossen 2011, Theorem 3.2
C12 = -skew(M(1:3,1:3) * nu(1:3));
C = [ zeros(3)   C12                        ;
    C12       -skew(M(4:6,4:6) * nu(4:6)) ];

% Construct damping matrix
D = -diag([Xu * abs(u), Yv * abs(v),...
    Zw * abs(w), Kp * abs(p),...
    Mq * abs(q), Nr * abs(r)]);

% Build state space equations
tau  = [ in(1); 0; 0; in(2:4) ];

dx       = zeros(12,1);
dx(1:6)  = J*nu;
dx(7:12) = M \ (tau - (C+D)*nu - G);
end

function S = skew(lambda)
S = [  0          -lambda(3)   lambda(2) ;
    lambda(3)   0          -lambda(1) ;
    -lambda(2)   lambda(1)   0         ];
end

function R = body_frame_rotation(Phi)
phi = Phi(1); theta = Phi(2); psi = Phi(3);

R = [  cos(psi)*cos(theta)  cos(psi)*sin(theta)*sin(phi)-sin(psi)*cos(phi)  cos(psi)*cos(phi)*sin(theta)+sin(psi)*sin(phi) ;
    sin(psi)*cos(theta)  sin(psi)*sin(theta)*sin(phi)+cos(psi)*cos(phi)  sin(psi)*cos(phi)*sin(theta)-cos(psi)*sin(phi) ;
    -sin(theta)           cos(theta)*sin(phi)                             cos(theta)*cos(phi)                            ];
end

== matlab function simulation_Hippocampus_compare_paper/Stabilizing without v w 1/HippCampus/MATLAB Function ==
  data: u input; y output
function y = fcn(u)
v = 0;
w = 0;
y = [u(1:7);v;w;u(10:12)];

== matlab function simulation_Hippocampus_compare_paper/Stabilizing without v w 1/HippCampus/Subsystem/MATLAB Function ==
  data: u input; y output
function y = fcn(u)
y =  wrapToPi(u);

== matlab function simulation_Hippocampus_compare_paper/Stabilizing without v w 1/HippCampus/Subsystem1/norm1 ==
  data: u input; y output
function y  = fcn(u)
y=norm(u)^2;
end

== matlab function simulation_Hippocampus_compare_paper/Stabilizing without v w 1/HippCampus/Subsystem4/Subsystem/norm1 ==
  data: u input; y output
function y  = fcn(u)
y=norm(u)^2;
end

== matlab function simulation_Hippocampus_compare_paper/Stabilizing without v w 1/HippCampus/Subsystem4/Subsystem1/norm1 ==
  data: u input; y output
function y  = fcn(u)
y=norm(u)^2;
end

== matlab function simulation_Hippocampus_compare_paper/Stabilizing without v w 1/HippCampus/Subsystem4/Subsystem2/norm1 ==
  data: u input; y output
function y  = fcn(u)
y=norm(u)^2;
end

== matlab function simulation_Hippocampus_compare_paper/Proposed nonlinear gain/HippCampus/sat1 ==
  data: u input; u_sat output; omega output
function [u_sat, omega] = fcn(u)
  %  u_sat=u;
    h     = 0.0481;   % [m] Distance of rotors to HippoCampus center
    Cd    = 0.0024;   % Coefficient of drag for the rotors
    tlim  = 3;        % Maximal torque of the motors 

    Q = [1,1,1,1;-Cd,Cd,-Cd,Cd;-h,-h,h,h;h,-h,-h,h];
    Qinv = inv(Q);

    % Transform into rotor space
    omega = Qinv*u;

    % Calculate utilization of each rotor
    util  = abs(omega/tlim);

    % Saturate torque at max utilization
    omega = omega ./ max(util, 1);    

    %Transform back into body frame
   u_sat = Q * omega;
end

== matlab function simulation_Hippocampus_compare_paper/Stabilizing without v w 1/HippCampus/Subsystem4/Subsystem3/norm1 ==
  data: u input; y output
function y  = fcn(u)
y=norm(u)^2;
end

== matlab function simulation_Hippocampus_compare_paper/Stabilizing without v w 1/HippCampus/sat1 ==
  data: u input; u_sat output; omega output
function [u_sat, omega] = fcn(u)
  %  u_sat=u;
    h     = 0.0481;   % [m] Distance of rotors to HippoCampus center
    Cd    = 0.0024;   % Coefficient of drag for the rotors
    tlim  = 3;        % Maximal torque of the motors 

    Q = [1,1,1,1;-Cd,Cd,-Cd,Cd;-h,-h,h,h;h,-h,-h,h];
    Qinv = inv(Q);

    % Transform into rotor space
    omega = Qinv*u;

    % Calculate utilization of each rotor
    util  = abs(omega/tlim);

    % Saturate torque at max utilization
    omega = omega ./ max(util, 1);    

    %Transform back into body frame
   u_sat = Q * omega;
end

== matlab function simulation_Hippocampus_compare_paper/Subsystem4/MATLAB Function3 ==
  data: u input; y output
function y = fcn(u)
y = sqrt(u(1)^2+u(2)^2+u(3)^2);

== matlab function simulation_Hippocampus_compare_paper/Subsystem4/MATLAB Function6 ==
  data: u input; y output
function y = fcn(u)
y =(u(1)^2+u(2)^2+u(3)^2);

== matlab function simulation_Hippocampus_compare_paper/Subsystem5/MATLAB Function3 ==
  data: u input; y output
function y = fcn(u)
y = sqrt(u(1)^2+u(2)^2+u(3)^2);

== matlab function simulation_Hippocampus_compare_paper/Subsystem5/MATLAB Function6 ==
  data: u input; y output
function y = fcn(u)
y =(u(1)^2+u(2)^2+u(3)^2);

== matlab function simulation_Hippocampus_compare_paper/Subsystem6/MATLAB Function3 ==
  data: u input; y output
function y = fcn(u)
y = sqrt(u(1)^2+u(2)^2+u(3)^2);

== matlab function simulation_Hippocampus_compare_paper/Subsystem6/MATLAB Function6 ==
  data: u input; y output
function y = fcn(u)
y =(u(1)^2+u(2)^2+u(3)^2);

== matlab function simulation_Hippocampus_compare_paper/Proposed nonlinear gain2/Controller/Passive Sigma3 ==
  data: s input; Theta_d input; omega_f output; Q3 input
%---------------------------------------------------------------------------------------------
% For Paper, 
% "Three-Dimensional Simultaneous Stabilization and Tracking Control of Nonholonomic Autonomous Underwater Vehicles"
% by Shuyuan Fan and Herbert Werner
% Copyright (c) Institute of Control Systems, Hamburg University of Technology. All rights reserved.
% Licensed under the GPLv3. See LICENSE in the project root for license information.
% Uses an own implementation of the work of 
% IEEE Conference on Decision and Control and L-CSS, 2022."
% Author(s): Shuyuan Fan
%--------------------------------------------------------------------------------------------
function omega_f= fcn(s,Theta_d,Q3)

%% states
x = s(1); y = s(2); z = s(3);
X = s(1:3);

angle = s(4:6);
phi = s(4);
%phi =min(max(phi,-0.5),0.5);
theta = s(5); 
%theta = min(max(theta,-1.5),1.5);
psi = s(6);
%psi =  wrapToPi(psi);
nu = s(7:9) ;
u=s(7); v=s(8); w=s(9); 

omega = s(10:12);
p=s(10); q=s(11); r=s(12);

% storage function V3
V3 = 0.5*(angle-Theta_d)'*(angle-Theta_d);

T = Jaco(angle);

y3star = angle-Theta_d;
omega_f = inv(T)*(Q3*y3star);


end

== matlab function simulation_Hippocampus_compare_paper/Proposed nonlinear gain2/Controller/Passive Sigma4 ==
  data: s input; omega_f input; tau2 output; Q4 input
%---------------------------------------------------------------------------------------------
% For Paper, 
% "Three-Dimensional Simultaneous Stabilization and Tracking Control of Nonholonomic Autonomous Underwater Vehicles"
% by Shuyuan Fan and Herbert Werner
% Copyright (c) Institute of Control Systems, Hamburg University of Technology. All rights reserved.
% Licensed under the GPLv3. See LICENSE in the project root for license information.
% Uses an own implementation of the work of 
% IEEE Conference on Decision and Control and L-CSS, 2022."
% Author(s): Shuyuan Fan
%--------------------------------------------------------------------------------------------
function tau2= fcn(s,omega_f,Q4)
zg    =  0.05;    % [m]
g     =  9.81;    % [m/s^2]

m     =  1.43;    % [kg]
Ix    = 0.00241; % [kgm^2]
Iy    = 0.01072; % [kgm^2]
Iz    = 0.01072; % [kgm^2]
Xudot = -1.11;    % [kg]
Yvdot = -2.80;    % [kg]
Zwdot = -2.80;    % [kg]
Kpdot = -0.0018;  % [kgm^2]
Mqdot = -0.0095;  % [kgm^2]
Nrdot = -0.0095;  % [kgm^2]
Xu    = -4.56;    % [kg/m]
Yv    = -17.36;   % [kg/m]
Zw    = -17.36;   % [kg/m]
Kp    = -0.0028;  % [kgm^2]
Mq    = -0.0476;  % [kgm^2]
Nr    = -0.0476;  % [kgm^2]

% Calculate mass matrix
Ma  = -diag([Xudot, Yvdot, Zwdot, Kpdot, Mqdot, Nrdot]);
Mrb =  diag([m,  m,  m, Ix, Iy, Iz]);
M = Ma + Mrb;

M1 = M(1:3,1:3);
M2 = M(4:6,4:6);



%% states
x = s(1); y = s(2); z = s(3);
X = s(1:3);

angle = s(4:6);
phi = s(4);
%phi =min(max(phi,-0.5),0.5);
theta = s(5); 
%theta = min(max(theta,-1.5),1.5);
psi = s(6);
%psi =  wrapToPi(psi);
nu = s(7:9) ;
u=s(7); v=s(8); w=s(9); 

omega = s(10:12);
p=s(10); q=s(11); r=s(12);


% Gamma function for nu
Gamma_nu = vectortodirect(nu);

y4 = omega;
y4star = y4 - omega_f;
% storage function V2
V2 = 0.5*y2star'*Gamma_nu'*M1*M1*Gamma_nu*y2star;


C1 = -skew(M(1:3,1:3) * nu);
C2 = -skew(M(4:6,4:6) * omega);
D = -diag([Xu * abs(u), Yv * abs(v),...
    Zw * abs(w), Kp * abs(p),...
    Mq * abs(q), Nr * abs(r)]);
D1 = D(1:3,1:3);
D2 = D(4:6,4:6);
gravity = zg * g * m;
G = [ 0; 0; 0; gravity * cos(theta) * sin(phi); gravity * sin(theta); 0 ];
g2 = G(4:6);
O = -C1*nu-C2*omega-D2*omega-g2;
tau2 = inv(M2)*(Q4*y4star-M2*O);

end

== matlab function simulation_Hippocampus_compare_paper/PDPD/norm ==
  data: u input; y output
function y  = fcn(u)
y=norm(u)^2;
end

== matlab function simulation_Hippocampus_compare_paper/Proposed nonlinear gain/Disturbance: All derivatives1/MATLAB Function1 ==
  data: u input; d output
function d = fcn(u)
z = u(3);
%a = mod(z,4); 
if z<2
      d =  [zeros(6,1);0.2*ones(6,1)];
elseif z<4
    d =  [zeros(6,1);0.4*ones(6,1)];
elseif z<6
    d =  [zeros(6,1);0.6*ones(6,1)];
elseif z<8
    d =  [zeros(6,1);0.8*ones(6,1)];
elseif z<10
    d =  [zeros(6,1);1*ones(6,1)];
else
    d=zeros(12,1);
end

% if a<3
%     d=zeros(12,1);
% else
%     d = [zeros(6,1);ones(6,1)];
% end

== matlab function simulation_Hippocampus_compare_paper/NDI/Disturbance: All derivatives2/MATLAB Function ==
  data: u input; y output; d input
function y = fcn(u,d)

y = u*d;

== matlab function simulation_Hippocampus_compare_paper/NDI/Disturbance: All derivatives2/MATLAB Function1 ==
  data: u input; d output
function d = fcn(u)
z = u(3);
a = mod(z,4); 
 
if a<3
    d=zeros(12,1);
else
    d = [zeros(6,1);ones(6,1)];
end

== matlab function simulation_Hippocampus_compare_paper/NDI/Disturbance: All derivatives2/disturbance3/MATLAB Function ==
  data: p input; a input; d output; u_wave input; u_c input; u_un input
%% wind disturbance, wave disturbance, ocean currents and modeling uncertainties(Fossen 2011)
%for AUV, we can neglect the wind disturbance
%wave disturbance is in R^6
%Ocean Currents are related to the hydrodynamic terms. Here we consider
%them as the friction forces 
%modeling uncertainties can be assumed as constant terms
%assume all disturbances are constant
function d = fcn(p,a,u_wave, u_c,u_un)
%a: attitude states
%u_wave: parameters of u_wave
%u_c ocean currents percentage
%u_un uncertainty percentage
%ocean currents
phi=a(1);
theta=a(2);
psi = a(3);
V = u_c(1)/100*4.724; % 0<V<4.724
theta_c=u_c(2);
psi_c = u_c(3);
 R = [  cos(psi)*cos(theta)  cos(psi)*sin(theta)*sin(phi)-sin(psi)*cos(phi)  cos(psi)*cos(phi)*sin(theta)+sin(psi)*sin(phi) ;
           sin(psi)*cos(theta)  sin(psi)*sin(theta)*sin(phi)+cos(psi)*cos(phi)  sin(psi)*cos(phi)*sin(theta)-cos(psi)*sin(phi) ;
          -sin(theta)           cos(theta)*sin(phi)                             cos(theta)*cos(phi)                            ];
uc=[V*cos(theta_c)*cos(psi_c);V*sin(psi_c);V*sin(theta_c)*cos(psi_c)];
f_c=R*uc;
d_c=[f_c;zeros(3,1)];

%wave disturbance
k1=u_wave(1:6); %amplitude 
k2 = u_wave(7:12); %frequency 
time=u_wave(13);
d_w = [k1(1)/100*4.724*sin(k2(1)*time);k1(2)/100*4.724*sin(k2(2)*time);k1(3)/100*4.724*sin(k2(3)*time);
    k1(4)/100*6.841*sin(k2(4)*time);k1(5)/100*28.55*sin(k2(5)*time);k1(6)/100*28.55*sin(k2(6)*time)];
%model uncertainties
%u_un uncertainty percentage
d_u=u_un/100*[4.724;0;0;6.841;28.55;28.55];

x=p(1);
y=p(2);
z=p(3);
if y>2 && y<2.5 || y<-2 && y>-2.5
    tau_d=d_c+d_w+d_u;
else
    tau_d=zeros(6,1);
end
    
d=[zeros(6,1);tau_d];

== matlab function simulation_Hippocampus_compare_paper/Proposed nonlinear gain/Controller/calculate derivative 1/MATLAB Function ==
  data: u input; y output; t input
function y = fcn(u,t)
if t>0.1
    y=u;
else
    y=[0;0;0;0];
end

== matlab function simulation_Hippocampus_compare_paper/Proposed Linear gain/Disturbance: All derivatives2/MATLAB Function1 ==
  data: u input; d output
function d = fcn(u)
z = u(3);
%a = mod(z,4); 
if z<2
      d =  [zeros(6,1);0.2*ones(6,1)];
elseif z<4
    d =  [zeros(6,1);0.4*ones(6,1)];
elseif z<6
    d =  [zeros(6,1);0.6*ones(6,1)];
elseif z<8
    d =  [zeros(6,1);0.8*ones(6,1)];
elseif z<10
    d =  [zeros(6,1);1*ones(6,1)];
else
    d=zeros(12,1);
end

% if a<3
%     d=zeros(12,1);
% else
%     d = [zeros(6,1);ones(6,1)];
% end

== matlab function simulation_Hippocampus_compare_paper/Proposed Linear gain/Disturbance: All derivatives2/disturbance3/MATLAB Function ==
  data: p input; a input; d output; u_wave input; u_c input; u_un input
%% wind disturbance, wave disturbance, ocean currents and modeling uncertainties(Fossen 2011)
%for AUV, we can neglect the wind disturbance
%wave disturbance is in R^6
%Ocean Currents are related to the hydrodynamic terms. Here we consider
%them as the friction forces 
%modeling uncertainties can be assumed as constant terms
%assume all disturbances are constant
function d = fcn(p,a,u_wave, u_c,u_un)
%a: attitude states
%u_wave: parameters of u_wave
%u_c ocean currents percentage
%u_un uncertainty percentage
%ocean currents
phi=a(1);
theta=a(2);
psi = a(3);
V = u_c(1)/100*4.724; % 0<V<4.724
theta_c=u_c(2);
psi_c = u_c(3);
 R = [  cos(psi)*cos(theta)  cos(psi)*sin(theta)*sin(phi)-sin(psi)*cos(phi)  cos(psi)*cos(phi)*sin(theta)+sin(psi)*sin(phi) ;
           sin(psi)*cos(theta)  sin(psi)*sin(theta)*sin(phi)+cos(psi)*cos(phi)  sin(psi)*cos(phi)*sin(theta)-cos(psi)*sin(phi) ;
          -sin(theta)           cos(theta)*sin(phi)                             cos(theta)*cos(phi)                            ];
uc=[V*cos(theta_c)*cos(psi_c);V*sin(psi_c);V*sin(theta_c)*cos(psi_c)];
f_c=R*uc;
d_c=[f_c;zeros(3,1)];

%wave disturbance
k1=u_wave(1:6); %amplitude 
k2 = u_wave(7:12); %frequency 
time=u_wave(13);
d_w = [k1(1)/100*4.724*sin(k2(1)*time);k1(2)/100*4.724*sin(k2(2)*time);k1(3)/100*4.724*sin(k2(3)*time);
    k1(4)/100*6.841*sin(k2(4)*time);k1(5)/100*28.55*sin(k2(5)*time);k1(6)/100*28.55*sin(k2(6)*time)];
%model uncertainties
%u_un uncertainty percentage
d_u=u_un/100*[4.724;0;0;6.841;28.55;28.55];

x=p(1);
y=p(2);
z=p(3);
if y>2 && y<2.5 || y<-2 && y>-2.5
    tau_d=d_c+d_w+d_u;
else
    tau_d=zeros(6,1);
end
    
d=[zeros(6,1);tau_d];

== matlab function simulation_Hippocampus_compare_paper/NDI4/Controller/MATLAB Function ==
  data: theta_des input; theta_des output; x input
function theta_des = fcn(theta_des, x)
yaw = x(6);
yaw_des = theta_des(3);
e_yaw = yaw_des-yaw;

% jump from -pi to +pi
if (e_yaw > pi)
    yaw_des = yaw_des - 2*pi;
% jump from +pi to -pi
elseif (-e_yaw > pi)
    yaw_des = yaw_des + 2*pi;
end
theta_des(3) = yaw_des;

== matlab function simulation_Hippocampus_compare_paper/NDI4/Controller/Pos controller1 ==
  data: r input; x input; u output; theta_des output; k_pos input; k_vel input
function [u,theta_des] = fcn(r, x,k_pos,k_vel)
%% Heuristic position controller
% Just wrap around a hueristic position controller around the attitude
% controller
%
% Gains that work for backup
% k_pos=2;
% k_vel=2;

drive_forward=1; % Easier to drive the unicycle backward than forward
if drive_forward==1
    e=r(1:3,1)-x(1:3,1);
    v_des=k_pos*norm(e,2);
else
    e=x(1:3,1)-r(1:3,1);
    v_des=-k_pos*norm(e,2);    
end
u=k_vel*(v_des-x(4));
proj_dist_xy=norm(e(1:2,1),2);
pitch_des=-atan2(e(3,1),proj_dist_xy);
psi_des=atan2(e(2),e(1));
theta_des=[0;pitch_des;psi_des]; 
end
